simulink model "Debug_LQR_Copy"  (R2016b)
settings: Solver=VariableStepAuto  StartTime=0.0  StopTime=30  RelTol=1e-3
undefined symbols (not defined in the file): adinchannels, adinchannelsencoders, adingain, adingainencoders, adinoffs, adinoffsencoders, Ao, Bo, Co, daoutchannels, daoutgain, daoutoffs, F, h, Humusoft, L, MF634, RefFWD, sigbuilder_block, xinit
libraries: sldrtlib x3, simulink x2, dspfdesign x1
settings Model: Creator=tcbooij  LastModifiedBy=tcbooij

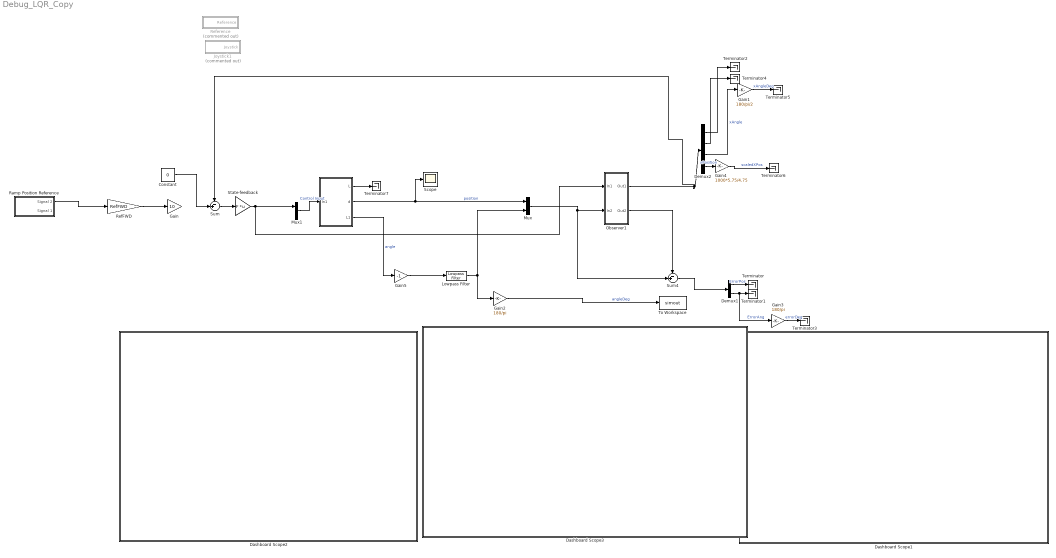
== system Debug_LQR_Copy ==
  " " : Subsystem  LoadFcn=hwinit  InitFcn=hwinit  mask{h=h}
      mask prompts: h "Sampling period [s]"
      mask Display: disp('Crane')
  Constant : Constant  Value=0
  Dashboard Scope1 : Subsystem  DialogController=hmiCreateDDGDialog  IsWebBlock=on  mask(MWDashboardBlock){webBlockId=94ce42f8-c4e1-41da-82c1-a31c02963333, webBlockType=sdiscope, ShowInitialText=on, HMISrcModelName=Debug_LQR_Copy}
      mask prompts: webBlockId "WebBlock Id"; webBlockType "WebBlock Type"; HMISrcModelName "Source Model"
      mask help: SimulinkHMI:dialogs:HMIScopeDialogDesc
      mask Help: helpview([docroot '/mapfiles/simulink.map'], 'hmi_scope')
      mask Display:
      | if strcmp(get_param(bdroot(gcb),'BlockDiagramType'), 'library')
      |     image([(matlabroot) '/toolbox/simulink/hmi/icons/DashboardScope.png']);
      | end
  Dashboard Scope2 : Subsystem  DialogController=hmiCreateDDGDialog  IsWebBlock=on  mask(MWDashboardBlock){webBlockId=2571b827-ae84-4a1c-bc36-e22ee194435d, webBlockType=sdiscope, ShowInitialText=on, HMISrcModelName=Debug_LQR_Copy}
      mask prompts: webBlockId "WebBlock Id"; webBlockType "WebBlock Type"; HMISrcModelName "Source Model"
      mask help: SimulinkHMI:dialogs:HMIScopeDialogDesc
      mask Help: helpview([docroot '/mapfiles/simulink.map'], 'hmi_scope')
      mask Display:
      | if strcmp(get_param(bdroot(gcb),'BlockDiagramType'), 'library')
      |     image([(matlabroot) '/toolbox/simulink/hmi/icons/DashboardScope.png']);
      | end
  Dashboard Scope3 : Subsystem  DialogController=hmiCreateDDGDialog  IsWebBlock=on  mask(MWDashboardBlock){webBlockId=8652e169-738a-43eb-99bc-869d98056901, webBlockType=sdiscope, ShowInitialText=on, HMISrcModelName=Debug_LQR_Copy}
      mask prompts: webBlockId "WebBlock Id"; webBlockType "WebBlock Type"; HMISrcModelName "Source Model"
      mask help: SimulinkHMI:dialogs:HMIScopeDialogDesc
      mask Help: helpview([docroot '/mapfiles/simulink.map'], 'hmi_scope')
      mask Display:
      | if strcmp(get_param(bdroot(gcb),'BlockDiagramType'), 'library')
      |     image([(matlabroot) '/toolbox/simulink/hmi/icons/DashboardScope.png']);
      | end
  Demux1 : Demux  Outputs=2
  Demux2 : Demux
  Gain : Gain  Gain=10
  Gain1 : Gain  Gain=180/pi/2
  Gain2 : Gain  Gain=180/pi
  Gain3 : Gain  Gain=180/pi
  Gain4 : Gain  Gain=1000*5.75/4.75
  Gain5 : Gain  Gain=-1
  Joystick1 : Subsystem  Commented=on
      mask Display: disp('Joystick')
  Lowpass Filter : dspfdesign/Lowpass Filter  FilterType=IIR  DesignForMinimumOrder=on  FilterOrder=50  PassbandFrequency=1e2  StopbandFrequency=2e2  PassbandRipple=0.1  StopbandAttenuation=80  InheritSampleRate=off  SampleRate=44100  SimulateUsing=Interpreted execution  roundingMode=Floor  coeffsDataTypeStr=fixdt(1,16)
  Mux : Mux  Inputs=2
  Mux1 : Mux  Inputs=2
  Observer1 : Subsystem
  Ramp Position Reference : Subsystem  Tag=STV Subsys  LoadFcn=sigbuilder_block('load');  StartFcn=sigbuilder_block('start');  StopFcn=sigbuilder_block('stop');  ClipboardFcn=sigbuilder_block('clipboard');  mask(Sigbuilder block){tuvar=[0:10]}
      mask help: Simulink:masks:SigbuilderBlock_MD
      mask init:
      | if ~strcmp(get_param(bdroot(gcbh),'SimulationStatus'),'stopped') tuvar = sigbuilder_block('maskInit'); end
      settings: CopyFcn=sigbuilder_block('copy');  DeleteFcn=sigbuilder_block('delete');  ModelCloseFcn=sigbuilder_block('modelClose');  PreSaveFcn=sigbuilder_block('preSave');  PauseFcn=sigbuilder_block('pause');  ContinueFcn=sigbuilder_block('continue');  NameChangeFcn=sigbuilder_block('namechange');  OpenFcn=sigbuilder_block('open',[403.5 83.25 565.5 401.25 ]);  CloseFcn=sigbuilder_block('close');
      mask Display: plot(0, 0, 100, 100,[2, 2, 32, 32, 2], [68, 8, 8, 68, 68],[32, 2], [38, 38], [32, 19, 2],[53, 60, 44], [32, 17, 17, 2],[16, 16, 31, 31]);txt = getActiveGroup(gcbh);text(2, 100, txt,'verticalAlignment', 'top');
  RefFWD : Gain  Gain=RefFWD
  Reference : Subsystem  Commented=on
      mask Display: disp('Reference')
  Scope : Scope
  State-feedback : Gain  Gain=F  Multiplication=Matrix(K*u)
  Sum : Sum  Inputs=-+|
  Sum4 : Sum  Inputs=-+|
  Terminator{,1..7} (8 alike) : Terminator
  To Workspace : ToWorkspace  VariableName=simout  SaveFormat=Timeseries  SampleTime=-1
  wires:
  Demux1/2 -> Gain3/1, Terminator1/1  "ErrorAng"
  Demux1/1 -> Terminator/1  "ErrorPos"
  Gain2/1 -> To Workspace/1  "angleDeg"
  Gain3/1 -> Terminator3/1  "errorDeg"
  " "/3(L1) -> Gain5/1  "angle"
  " "/2(d) -> Mux/1, Scope/1  "position"
  State-feedback/1 -> Observer1/1(In1), Mux1/1
  Sum4/1 -> Demux1/1
  Demux2/4 -> Gain4/1  "xPosition"
  Demux2/3 -> Gain1/1  "xAngle"
  Demux2/2 -> Terminator4/1
  Demux2/1 -> Terminator2/1
  Gain1/1 -> Terminator5/1  "xAngleDeg"
  Gain4/1 -> Terminator6/1  "scaledXPos"
  RefFWD/1 -> Gain/1
  Sum/1 -> State-feedback/1
  Lowpass Filter/1 -> Gain2/1, Mux/2
  Mux1/1 -> " "/1(In1)  "Control Input"
  " "/1(L) -> Terminator7/1
  Mux/1 -> Sum4/2, Observer1/2(In2)
  Ramp Position Reference/1(Signal 2) -> RefFWD/1
  Constant/1 -> Sum/2
  Gain5/1 -> Lowpass Filter/1
  Observer1/1(Out1) -> Sum/1, Demux2/1
  Observer1/2(Out2) -> Sum4/1

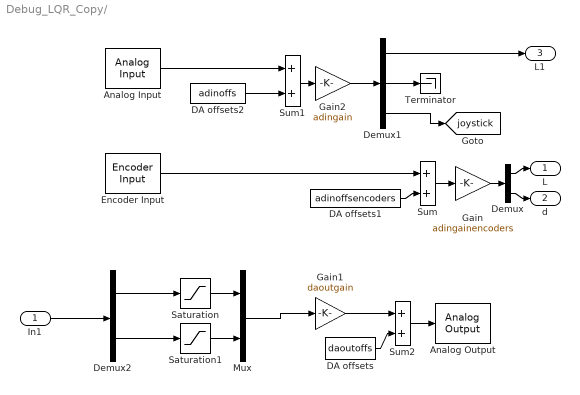
== system Debug_LQR_Copy/  ==
  In1 : Inport
  Analog Input : sldrtlib/Analog Input  SampleTime=h  MaxMissedTicks=ticklost  ShowMissedTicks=off  YieldWhenWaiting=off  DrvName=Humusoft/MF634  DrvAddress=4294967295  DrvOptions=0  Channels=[adinchannels]  RangeMode=2  VoltRange=1  DataType=1
      settings: AttributesFormatString=Humusoft\nMF634 [auto]
  Analog Output : sldrtlib/Analog Output  SampleTime=h  MaxMissedTicks=ticklost  ShowMissedTicks=off  YieldWhenWaiting=off  DrvName=Humusoft/MF634  DrvAddress=4294967295  DrvOptions=0  Channels=[daoutchannels]  RangeMode=2  VoltRange=1  InitialValue=0  FinalValue=0
      settings: AttributesFormatString=Humusoft\nMF634 [auto]
  DA offsets : Constant  Value=daoutoffs
  DA offsets1 : Constant  Value=adinoffsencoders
  DA offsets2 : Constant  Value=adinoffs
  Demux : Demux  Outputs=2
  Demux1 : Demux  Outputs=[1 1 2]
  Demux2 : Demux  Outputs=2
  Encoder Input : sldrtlib/Encoder Input  SampleTime=h  MaxMissedTicks=ticklost  ShowMissedTicks=off  YieldWhenWaiting=off  DrvName=Humusoft/MF634  DrvAddress=4294967295  DrvOptions=0  Channels=[adinchannelsencoders]  QuadMode=3  IndexPulse=1  InputFilter=Inf  DataType=1
      settings: AttributesFormatString=Humusoft\nMF634 [auto]
  Gain : Gain  Gain=adingainencoders  SaturateOnIntegerOverflow=on  OutDataTypeStr=Inherit: Same as input  ParamDataTypeStr=Inherit: Same as input
  Gain1 : Gain  Gain=daoutgain  SaturateOnIntegerOverflow=on  OutDataTypeStr=Inherit: Same as input  ParamDataTypeStr=Inherit: Same as input
  Gain2 : Gain  Gain=adingain  SaturateOnIntegerOverflow=on  OutDataTypeStr=Inherit: Same as input  ParamDataTypeStr=Inherit: Same as input
  Mux : Mux  Inputs=2
  Saturation : Saturate  UpperLimit=10  LowerLimit=-10
  Saturation1 : Saturate  UpperLimit=10  LowerLimit=-10
  Sum : Sum  SaturateOnIntegerOverflow=on  InputSameDT=on  OutDataTypeStr=Inherit: Same as first input
  Sum1 : Sum  SaturateOnIntegerOverflow=on  InputSameDT=on  OutDataTypeStr=Inherit: Same as first input
  Sum2 : Sum  SaturateOnIntegerOverflow=on  InputSameDT=on  OutDataTypeStr=Inherit: Same as first input
  Terminator : Terminator
  L : Outport  Tag=Position
  d : Outport  Tag=Cable length  Port=2
  L1 : Outport  Tag=Position  Port=3
  tag scope: joystick=global
  wires:
  Gain/1 -> Demux/1
  Sum/1 -> Gain/1
  DA offsets1/1 -> Sum/2
  Sum1/1 -> Gain2/1
  Analog Input/1 -> Sum1/1
  DA offsets2/1 -> Sum1/2
  Demux/1 -> L/1
  Demux/2 -> d/1
  Gain2/1 -> Demux1/1
  Demux1/3 -> [joystick]
  Demux1/1 -> L1/1
  Gain1/1 -> Sum2/1
  Sum2/1 -> Analog Output/1
  DA offsets/1 -> Sum2/2
  Encoder Input/1 -> Sum/1
  In1/1 -> Demux2/1
  Demux2/1 -> Saturation/1
  Demux2/2 -> Saturation1/1
  Saturation/1 -> Mux/1
  Mux/1 -> Gain1/1
  Saturation1/1 -> Mux/2
  Demux1/2 -> Terminator/1

== system Debug_LQR_Copy/Dashboard Scope1 ==

== system Debug_LQR_Copy/Dashboard Scope2 ==

== system Debug_LQR_Copy/Dashboard Scope3 ==

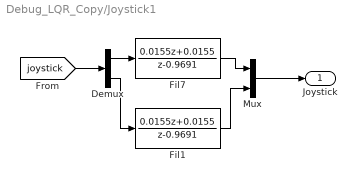
== system Debug_LQR_Copy/Joystick1 ==
  Demux : Demux  Outputs=2
  Fil1 : DiscreteTransferFcn  Numerator=[0.0155 0.0155]  Denominator=[1 -0.9691]  SampleTime=h
  Fil7 : DiscreteTransferFcn  Numerator=[0.0155 0.0155]  Denominator=[1 -0.9691]  SampleTime=h
  Mux : Mux  Inputs=2
  Joystick : Outport
  wires:
  Mux/1 -> Joystick/1
  Fil1/1 -> Mux/2
  Demux/2 -> Fil1/1
  Demux/1 -> Fil7/1
  [joystick] -> Demux/1
  Fil7/1 -> Mux/1

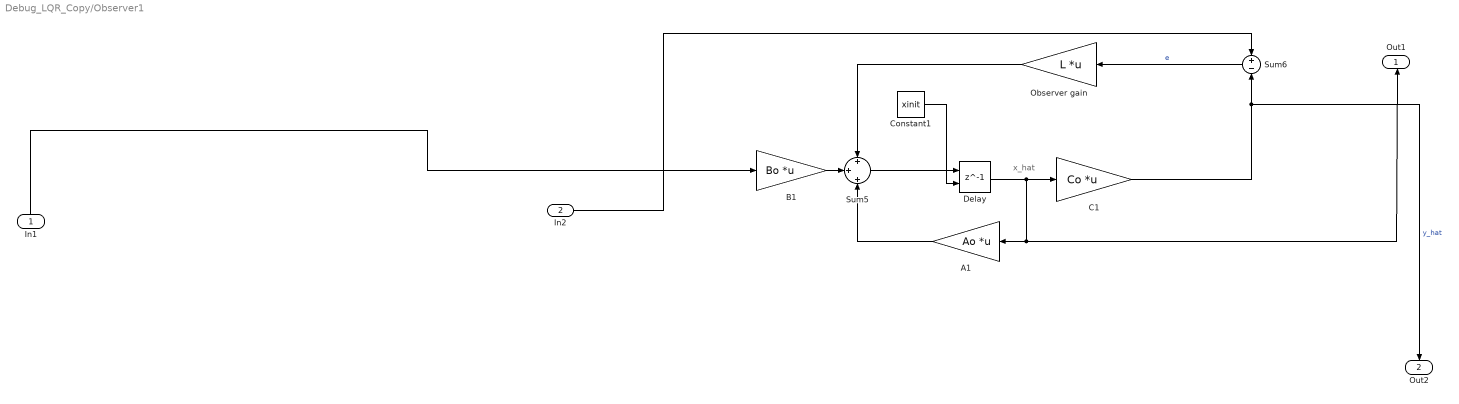
== system Debug_LQR_Copy/Observer1 ==
  note: x_hat
  In1 : Inport
  In2 : Inport  Port=2
  A1 : Gain  Gain=Ao  Multiplication=Matrix(K*u)
  B1 : Gain  Gain=Bo  Multiplication=Matrix(K*u)
  C1 : Gain  Gain=Co  Multiplication=Matrix(K*u)
  Constant1 : Constant  Value=xinit
  Delay : Delay  DelayLength=1  InitialConditionSource=Input port
      settings: InputPortMap=u0,p4
  Observer gain : Gain  Gain=L  Multiplication=Matrix(K*u)
  Sum5 : Sum  Inputs=+|+|+
  Sum6 : Sum  Inputs=+|-
  Out1 : Outport
  Out2 : Outport  Port=2
  wires:
  In2/1 -> Sum6/1
  In1/1 -> B1/1
  Delay/1 -> C1/1, Out1/1, A1/1
  Sum6/1 -> Observer gain/1  "e"
  A1/1 -> Sum5/3
  B1/1 -> Sum5/2
  C1/1 -> Out2/1, Sum6/2  "y_hat"
  Observer gain/1 -> Sum5/1
  Sum5/1 -> Delay/1
  Constant1/1 -> Delay/2

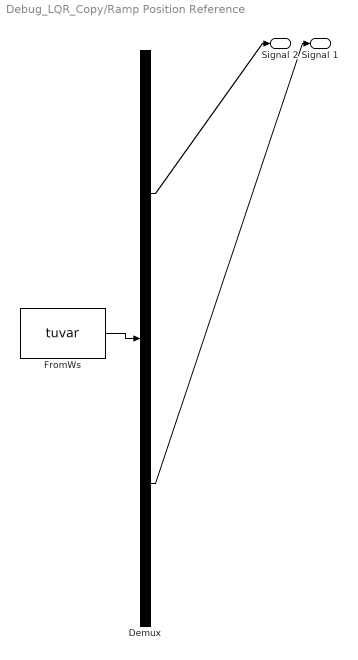
== system Debug_LQR_Copy/Ramp Position Reference ==
  Demux : Demux  Tag=STV Demux  Outputs=2
  FromWs : FromWorkspace  Tag=STV FromWs  VariableName=tuvar  SampleTime=0
      SigBuilderData=|
      | common.afterFinalStr = 'Extrapolate'
      | common.sampleTime = 0
      | dataSet.timeRange = [0 30]
      | dataSet.name = 'Group 1'
      | sbobj.Groups.Name = 'Group 1'
      | sbobj.Groups.Signals(1).Name = 'Signal 2'
      | sbobj.Groups.Signals(1).XData = [0 2.5 5 7.5 10 12.5 15 17.5 20 22.5 25 27.5 30]
      | sbobj.Groups.Signals(1).YData = [0 0 1 1 0 0 -1 -1 0 0 1 1 0]
      | sbobj.Groups.Signals(2).Name = 'Signal 1'
      | sbobj.Groups.Signals(2).XData = [0 0.0408163265306 0.0816326530612 0.122448979592 0.163265306122 0.204081632653 0.244897959184 0.285714285714 0.326530612245 0.367346938776 0.408163265306 0.448979591837 ... (736 elements, 1x736)]
      | sbobj.Groups.Signals(2).YData = [0 0.255754323369 0.507309167819 0.750534009759 0.981435104008 1.19622106098 1.39136510121 1.56366296494 1.71028552601 1.82882524603 1.91733570607 1.97436356683 ... (736 elements, 1x736)]
      | sbobj.Groups.TimeRange = [0 30]
  Signal 2 : Outport  Tag=STV Outport
  Signal 1 : Outport  Tag=STV Outport  Port=2
  wires:
  FromWs/1 -> Demux/1
  Demux/1 -> Signal 2/1
  Demux/2 -> Signal 1/1

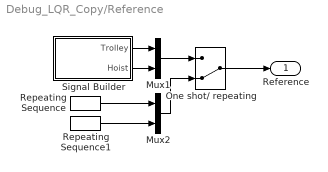
== system Debug_LQR_Copy/Reference ==
  Mux1 : Mux  Inputs=2
  Mux2 : Mux  Inputs=2
  One shot/ repeating : ManualSwitch  CurrentSetting=0
  Repeating Sequence : simulink/Sources/Repeating Sequence  rep_seq_t="[0    4.5000   12.5000   22.5000   30.5000   36.0000]"  rep_seq_y="[0         0    1.5000    1.5000         0         0]"
  Repeating Sequence1 : simulink/Sources/Repeating Sequence  rep_seq_t="[0     2     7    10    15    20    25    28    33    36]"  rep_seq_y="[0         0   -0.8000   -0.8000    0.3400    0.3400   -0.8000  -0.8000         0         0]"
  Signal Builder : Subsystem  Tag=STV Subsys  LoadFcn=sigbuilder_block('load');  StartFcn=sigbuilder_block('start');  StopFcn=sigbuilder_block('stop');  ClipboardFcn=sigbuilder_block('clipboard');  mask(Sigbuilder block){tuvar=[0:10]}
      mask help: Sigbuilder GUI
      mask init:
      | if ~strcmp(get_param(bdroot(gcb),'SimulationStatus'),'stopped') tuvar = sigbuilder_block('maskInit'); end
      settings: CopyFcn=sigbuilder_block('copy');  DeleteFcn=sigbuilder_block('delete');  ModelCloseFcn=sigbuilder_block('modelClose');  PreSaveFcn=sigbuilder_block('preSave');  PauseFcn=sigbuilder_block('pause')  ContinueFcn=sigbuilder_block('continue')  NameChangeFcn=sigbuilder_block('namechange');  OpenFcn=sigbuilder_block('open',[50.25 82.5 519.75 399.75 ]);  CloseFcn=sigbuilder_block('close');
      mask Display: plot(0, 0, 100, 100,[2, 2, 32, 32, 2], [68, 8, 8, 68, 68],[32, 2], [38, 38], [32, 19, 2],[53, 60, 44], [32, 17, 17, 2],[16, 16, 31, 31]);txt = getActiveGroup(gcbh);text(2, 100, txt,'verticalAlignment', 'top');
  Reference : Outport
  wires:
  Repeating Sequence1/1 -> Mux2/2
  Mux2/1 -> One shot/ repeating/2
  Repeating Sequence/1 -> Mux2/1
  Mux1/1 -> One shot/ repeating/1
  One shot/ repeating/1 -> Reference/1
  Signal Builder/1(Trolley) -> Mux1/1
  Signal Builder/2(Hoist) -> Mux1/2

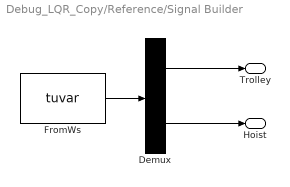
== system Debug_LQR_Copy/Reference/Signal Builder ==
  Demux : Demux  Tag=STV Demux  Outputs=2
  FromWs : FromWorkspace  Tag=STV FromWs  VariableName=tuvar  SampleTime=0
      SigBuilderData=|
      | dataSet.timeRange = [0 36]
      | dataSet.name = 'Group 1'
      | sbobj.Groups.Name = 'Group 1'
      | sbobj.Groups.Signals(1).Name = 'Trolley'
      | sbobj.Groups.Signals(1).XData = [0 4.5 12.5 22.5 30.5 36]
      | sbobj.Groups.Signals(1).YData = [0 0 1.5 1.5 0 0]
      | sbobj.Groups.Signals(2).Name = 'Hoist'
      | sbobj.Groups.Signals(2).XData = [0 2 7 10 15 20 25 28 33 36]
      | sbobj.Groups.Signals(2).YData = [0 0 -0.8 -0.8 0.34 0.34 -0.8 -0.8 0 0]
  Trolley : Outport  Tag=STV Outport
  Hoist : Outport  Tag=STV Outport  Port=2
  wires:
  Demux/2 -> Hoist/1
  Demux/1 -> Trolley/1
  FromWs/1 -> Demux/1
